simulink model "MODELLO_TURBINA_FUNZIONANTE"  (R2024a)
settings: Solver=VariableStepAuto  StartTime=0.0  StopTime=20  RelTol=1e-3
libraries: simulink x1
settings Model: Creator=emanuele  LastModifiedBy=emanuele

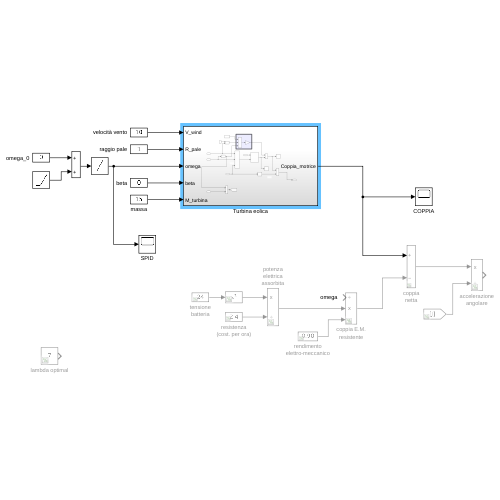
[thumbnail: Simulink's stored preview of the top-level diagram]
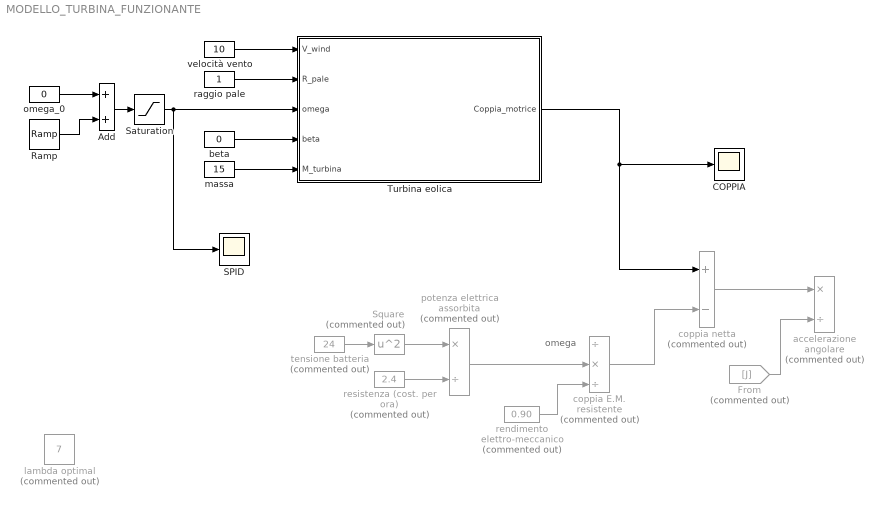
== system MODELLO_TURBINA_FUNZIONANTE ==
  note: omega
  Add : Sum
  COPPIA : Scope
  From : From  Commented=on  GotoTag=J
  Ramp : simulink/Sources/Ramp  slope=20  start=2  InitialOutput=0
  SPID : Scope
  Saturation : Saturate  UpperLimit=180  LowerLimit=1
  Square : Math  Commented=on  Operator=square
  Turbina eolica : Subsystem
  accelerazione angolare : Product  Commented=on  Inputs=*/
  beta : Constant  Value=0
  coppia netta : Sum  Commented=on  Inputs=+-
  coppia E.M. resistente : Product  Commented=on  Inputs=/*/
  lambda optimal : Constant  Commented=on  Value=7
  massa : Constant  Value=15
  omega_0 : Constant  Value=0
  potenza elettrica assorbita : Product  Commented=on  Inputs=*/
  raggio pale : Constant
  rendimento elettro-meccanico : Constant  Commented=on  Value=0.90
  resistenza (cost. per ora) : Constant  Commented=on  Value=2.4
  tensione batteria : Constant  Commented=on  Value=24
  velocità vento : Constant  Value=10
  wires:
  rendimento elettro-meccanico/1 -> coppia E.M. resistente/3
  tensione batteria/1 -> Square/1
  resistenza (cost. per ora)/1 -> potenza elettrica assorbita/2
  Square/1 -> potenza elettrica assorbita/1
  potenza elettrica assorbita/1 -> coppia E.M. resistente/2
  coppia E.M. resistente/1 -> coppia netta/2
  coppia netta/1 -> accelerazione angolare/1
  From/1 -> accelerazione angolare/2
  velocità vento/1 -> Turbina eolica/1(V_wind)
  raggio pale/1 -> Turbina eolica/2(R_pale)
  beta/1 -> Turbina eolica/4(beta)
  massa/1 -> Turbina eolica/5(M_turbina)
  Turbina eolica/1(Coppia_motrice) -> COPPIA/1, coppia netta/1
  omega_0/1 -> Add/1
  Add/1 -> Saturation/1
  Saturation/1 -> Turbina eolica/3(omega), SPID/1
  Ramp/1 -> Add/2

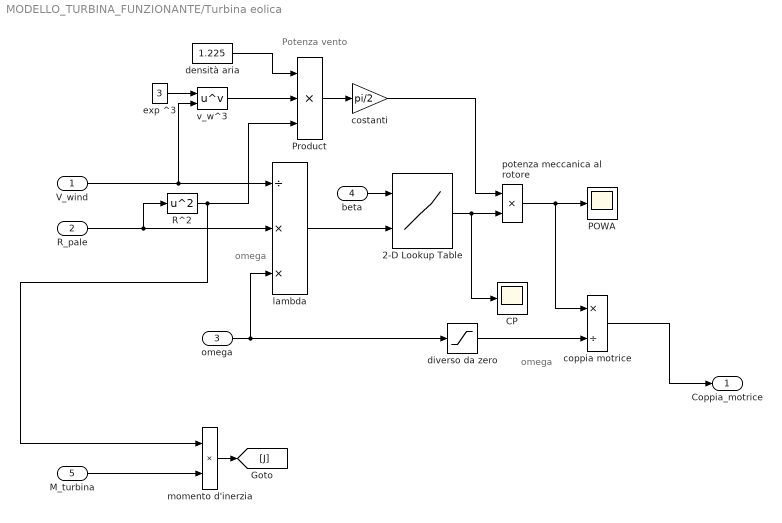
== system MODELLO_TURBINA_FUNZIONANTE/Turbina eolica ==
  note: Potenza vento
  note: omega
  note: omega
  V_wind : Inport
  R_pale : Inport  Port=2
  omega : Inport  Port=3
  beta : Inport  Port=4
  M_turbina : Inport  Port=5
  2-D Lookup Table : Lookup_n-D  BreakpointsForDimension1=[0, 3, 5, 10, 20, 90]  BreakpointsForDimension2=[0, 2, 4, 6, 8, 10, 12, 14, 15]  Table=[0.0010, 0.0161, 0.1446, 0.3865, 0.5009, 0.4404, 0.2545, 0.0002, -0.1384; 0.0016, 0.0173, 0.1079, 0.2676, 0.3779, 0.4111, 0.3838, 0.3176, 0.2753; 0.0027, 0.0197, 0.1151, 0.2606, 0.3469, 0.3558, 0.3069, 0.2222, 0.1718; 0.0054, 0.0283, 0.1315, 0.2364, 0.2589, 0.2022, 0.0929, -0.0455, -0.1204; 0.0109, 0.0536, 0.1320, 0.1256, 0.0120, -0.1752, -0.4017, -0.6435, -0.7655; -0.01 * ones(1, 9)]  InternalRulePriority=Speed  RndMeth=Simplest
      settings: InputPortMap=u0,u1
  CP : Scope
  POWA : Scope
  Product : Product  Inputs=***
  R^2 : Math  Operator=square
  coppia motrice : Product  Inputs=*/
  costanti : Gain  Gain=pi/2
  densità aria : Constant  Value=1.225
  diverso da zero : Saturate  UpperLimit=10e3  LowerLimit=0.1
  exp ^3 : Constant  Value=3
  lambda : Product  Inputs=/**
  momento d'inerzia : Product
  potenza meccanica al rotore : Product
  v_w^3 : Math  Operator=pow
  Coppia_motrice : Outport
  wires:
  potenza meccanica al rotore/1 -> POWA/1, coppia motrice/1
  coppia motrice/1 -> Coppia_motrice/1
  R_pale/1 -> lambda/2, R^2/1
  V_wind/1 -> v_w^3/2, lambda/1
  densità aria/1 -> Product/1
  v_w^3/1 -> Product/2
  costanti/1 -> potenza meccanica al rotore/1
  R^2/1 -> momento d'inerzia/1, Product/3
  exp ^3/1 -> v_w^3/1
  Product/1 -> costanti/1
  momento d'inerzia/1 -> [J]
  M_turbina/1 -> momento d'inerzia/2
  2-D Lookup Table/1 -> CP/1, potenza meccanica al rotore/2
  beta/1 -> 2-D Lookup Table/1
  lambda/1 -> 2-D Lookup Table/2
  omega/1 -> diverso da zero/1, lambda/3
  diverso da zero/1 -> coppia motrice/2
